simulink library "FuelSystemLibrary"  (R2014b)
settings: Solver=ode45  SolverMode=SingleTasking  StartTime=0.0  StopTime=10.0  RelTol=1e-3
undefined symbols (not defined in the file): BooleanOff, BooleanOn, BoolThreshold, BowserOnPressure, CouplingOffPressure, CouplingOnPressure, DefaultTemp, DiffuserResistance, DiscreteSwitchOff, DiscreteSwitchOn, DiscreteSwitchThreshold, FloatingPressure, FlowNoOverride, FspSamplingPeriod, FuelSpecificHeatCapacity, g, InfiniteFlow, InfiniteMass, InfiniteResistance, InfiniteTime, InfiniteVolume, kpl2kpm3, MaxAValue, MaxBValue, MeterNoReset, MinAValue, MinBValue, NearZeroMass, NearZeroTime, NoError, NominalAValue, NominalBValue, NonRetResistance, NoReset, NullBasePress, PerCycle2PerSec, PerSec2PerCycle, PipeDisconnected, PipeResistance, PumpOnTime, TankFixedMassError, TankInletResistance, TankInstPortStartOffset, TankNoReset, TypicalFuelDensity, ValveClosedPosition, ValveOnResistance, ValveOpenPosition, ValveOpenTime
libraries: FuelSystemLibrary x251, WrightSolverLib x50, simulink x1
(part 2 of 4)

== system FuelSystemLibrary/NRV_V2 ==
  note: No source available downstream,
      | no sink available upstream
  note: NRV: Simulation of Non Return Valve, using WrightSolver diode
      |
      | Revision History -
      | Issue 1.0 - 5th April 2011 - SW - Initial Issue
  BBBrk : FuelSystemLibrary/BBBrk
  BBBrk1 : FuelSystemLibrary/BBBrk1
  BBSrcBrk : FuelSystemLibrary/BBSrcBrk
  Constant2 : Constant  Value=0
  Diode_V2 : WrightSolverLib/Diode_V2
  SinkBrk : FuelSystemLibrary/BBSinkBrk
  Terminator3 : Terminator
  1P : PMIOPort  Tag=PMCPort  Port=1  Side=Left
  2P : PMIOPort  Tag=PMCPort  Port=2  Side=Right
  1BB : PMIOPort  Tag=PMCPort  Port=3  Side=Left
  2BB : PMIOPort  Tag=PMCPort  Port=4  Side=Right
  wires:
  Diode_V2/1 -> Terminator3/1
  Constant2/1 -> Diode_V2/1
  BBBrk1/1 -> SinkBrk/1
  SinkBrk/1 -> BBBrk/1
  BBBrk/1 -> BBSrcBrk/1
  BBSrcBrk/1 -> BBBrk1/1
  connections:
  1P/RConn1 -- Diode_V2/LConn1
  Diode_V2/RConn1 -- 2P/RConn1
  1BB/RConn1 -- BBBrk1/RConn1
  BBBrk/LConn1 -- 2BB/RConn1

== system FuelSystemLibrary/NumInPlug ==
  note: NumInPlug - Plug for numerical interface to tank
      |
      | Revision History -
      | Issue 1.0 - ?? - SW - Initial Issue
      | Issue 1.1 - 28th October 2005 - DR - Added to FSP Generic Library
  BBTerm : FuelSystemLibrary/BBTerm
  Constant : Constant  Value=0
  Terminator8 : Terminator
  Two-Way Connection1 : TwoWayConnection
  1P : PMIOPort  Tag=PMCPort  Port=1  Side=Right
  1BB : PMIOPort  Tag=PMCPort  Port=2  Side=Right
  wires:
  Two-Way Connection1/1 -> Terminator8/1
  Constant/1 -> Two-Way Connection1/1
  connections:
  Two-Way Connection1/RConn1 -- 1P/RConn1
  BBTerm/LConn1 -- 1BB/RConn1

== system FuelSystemLibrary/OFlowIface ==
  note: Translate crude Oflow interface into
      | numerical interface
  Oflow : Inport
  BBBrk : FuelSystemLibrary/BBBrk
  BBStub : FuelSystemLibrary/BBStub
  Demux6 : Demux  Outputs=2
  Terminator8 : Terminator
  Two-Way Connection1 : TwoWayConnection
  P : PMIOPort  Tag=PMCPort  Port=1  Side=Right
  BB : PMIOPort  Tag=PMCPort  Port=2  Side=Right
  wires:
  Demux6/2 -> BBBrk/1  "Info"
  Demux6/1 -> Two-Way Connection1/1  "Mass"
  Oflow/1 -> Demux6/1
  Two-Way Connection1/1 -> Terminator8/1
  BBBrk/1 -> BBStub/1
  connections:
  Two-Way Connection1/RConn1 -- P/RConn1
  BB/RConn1 -- BBBrk/LConn1

== system FuelSystemLibrary/OflowPlug ==
  BBNull : FuelSystemLibrary/BBNull
  Constant2 : Constant  Value=0
  P : Outport
  BB : Outport  Port=2
  wires:
  BBNull/1 -> BB/1
  Constant2/1 -> P/1

== system FuelSystemLibrary/Oriface ==
  C : Inport
  Delay : UnitDelay  InitialCondition=0.0  SampleTime=FspSamplingPeriod
  Delay1 : UnitDelay  InitialCondition=1000000.0  SampleTime=FspSamplingPeriod
  Res : WrightSolverLib/Res
  S-Function : S-Function  FunctionName=OrifaceControlBlockWrapper  EnableBusSupport=off
  2P : PMIOPort  Tag=PMCPort  Port=1  Side=Right
  1P : PMIOPort  Tag=PMCPort  Port=2  Side=Left
  1BB : PMIOPort  Tag=PMCPort  Port=3  Side=Left
  2BB : PMIOPort  Tag=PMCPort  Port=4  Side=Right
  wires:
  Res/1 -> Delay/1
  C/1 -> S-Function/2
  S-Function/1 -> Res/1, Delay1/1
  Delay/1 -> S-Function/1
  Delay1/1 -> S-Function/3
  connections:
  1P/RConn1 -- Res/LConn1
  Res/RConn1 -- 2P/RConn1
  1BB/RConn1 -- 2BB/RConn1

== system FuelSystemLibrary/Outlet ==
  note: outlet
      |
      | Revision History -
      | Issue 1.0 - ?? - SW - Initial Issue
      | Issue 1.1 - 28th October 2005 - DR - Added to FSP Generic Library
  note: Elevate the IO pressures
      | due to head pressures.
  note: We can assume that all tank outlets are connected to
      | pumps, thus ensuring that there can be no backflow
      | into the tank, or outflow if the outlet is not covered.
      |
      | Therefore no diode or cutoff switch, for maximum modelling efficiency.
  HeadPress : Inport
  PipeCovered : Inport  Port=2
  Constant12 : Constant  Value=FlowNoOverride
  I Tap : WrightSolverLib/I Tap
  Term : WrightSolverLib/Term
  Terminator : Terminator
  V : WrightSolverLib/V
  O1P : PMIOPort  Tag=PMCPort  Port=1  Side=Right
  Outflow : Outport
  wires:
  PipeCovered/1 -> Terminator/1
  [OutFlow] -> Outflow/1
  I Tap/1 -> [OutFlow]
  HeadPress/1 -> V/1
  Constant12/1 -> V/2, V/3
  connections:
  Term/RConn1 -- V/LConn1
  I Tap/RConn1 -- O1P/RConn1
  V/RConn1 -- I Tap/LConn1

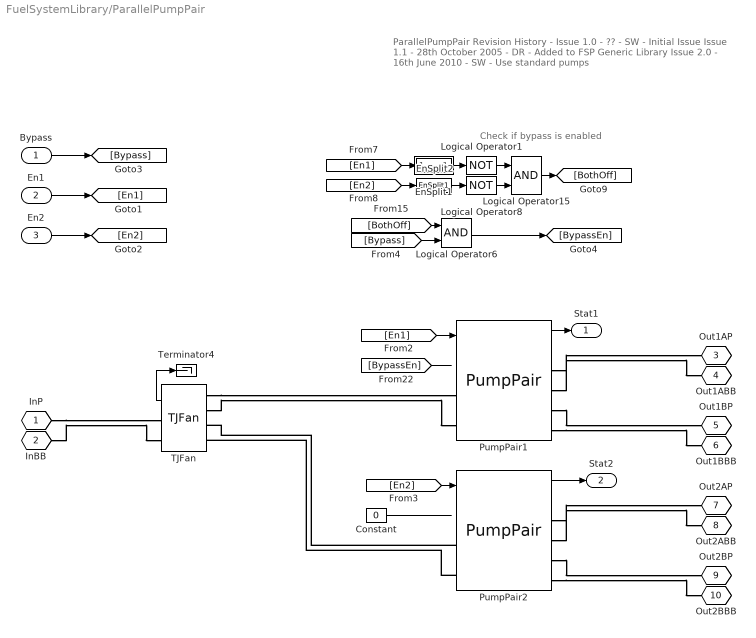
== system FuelSystemLibrary/ParallelPumpPair ==
  note: ParallelPumpPair
      |
      | Revision History -
      | Issue 1.0 - ?? - SW - Initial Issue
      | Issue 1.1 - 28th October 2005 - DR - Added to FSP Generic Library
      | Issue 2.0 - 16th June 2010 - SW - Use standard pumps
  note: Check if bypass is enabled
  Bypass : Inport
  En1 : Inport  Port=2
  En2 : Inport  Port=3
  Constant : Constant  Value=0
  EnSplit1 : Subsystem
  EnSplit2 : FuelSystemLibrary/ParallelPumpPair/EnSplit1
  Logical Operator1 : Logic  Operator=NOT  Inputs=3  AllPortsSameDT=off
  Logical Operator15 : Logic  AllPortsSameDT=off
  Logical Operator6 : Logic  AllPortsSameDT=off
  Logical Operator8 : Logic  Operator=NOT  Inputs=3  AllPortsSameDT=off
  PumpPair1 : FuelSystemLibrary/PumpPair
  PumpPair2 : FuelSystemLibrary/PumpPair
  TJFan : FuelSystemLibrary/TJFan
  Terminator4 : Terminator
  InP : PMIOPort  Tag=PMCPort  Port=1  Side=Left
  InBB : PMIOPort  Tag=PMCPort  Port=2  Side=Left
  Out1AP : PMIOPort  Tag=PMCPort  Port=3  Side=Right
  Out1ABB : PMIOPort  Tag=PMCPort  Port=4  Side=Right
  Out1BP : PMIOPort  Tag=PMCPort  Port=5  Side=Right
  Out1BBB : PMIOPort  Tag=PMCPort  Port=6  Side=Right
  Out2AP : PMIOPort  Tag=PMCPort  Port=7  Side=Right
  Out2ABB : PMIOPort  Tag=PMCPort  Port=8  Side=Right
  Out2BP : PMIOPort  Tag=PMCPort  Port=9  Side=Right
  Out2BBB : PMIOPort  Tag=PMCPort  Port=10  Side=Right
  Stat1 : Outport
  Stat2 : Outport  Port=2
  wires:
  TJFan/1 -> Terminator4/1
  Constant/1 -> ?
  [En1] -> PumpPair1/1
  PumpPair1/1 -> Stat1/1
  PumpPair2/1 -> Stat2/1
  [BypassEn] -> ?
  Bypass/1 -> [Bypass]
  [Bypass] -> Logical Operator6/2
  [BothOff] -> Logical Operator6/1
  Logical Operator15/1 -> [BothOff]
  Logical Operator8/1 -> Logical Operator15/2
  Logical Operator1/1 -> Logical Operator15/1
  EnSplit2/1 -> Logical Operator8/1
  Logical Operator6/1 -> [BypassEn]
  EnSplit1/1(On) -> Logical Operator1/1
  [En1] -> EnSplit1/1(En)
  [En2] -> EnSplit2/1
  En1/1 -> [En1]
  En2/1 -> [En2]
  [En2] -> PumpPair2/1
  connections:
  PumpPair2/LConn2 -- TJFan/LConn4
  PumpPair2/LConn1 -- TJFan/LConn3
  TJFan/LConn2 -- PumpPair1/LConn2
  TJFan/LConn1 -- PumpPair1/LConn1
  InBB/RConn1 -- TJFan/RConn2
  InP/RConn1 -- TJFan/RConn1
  PumpPair2/RConn2 -- Out2ABB/RConn1
  PumpPair2/RConn1 -- Out2AP/RConn1
  PumpPair2/RConn3 -- Out2BP/RConn1
  PumpPair2/RConn4 -- Out2BBB/RConn1
  PumpPair1/RConn1 -- Out1AP/RConn1
  PumpPair1/RConn2 -- Out1ABB/RConn1
  PumpPair1/RConn3 -- Out1BP/RConn1
  PumpPair1/RConn4 -- Out1BBB/RConn1

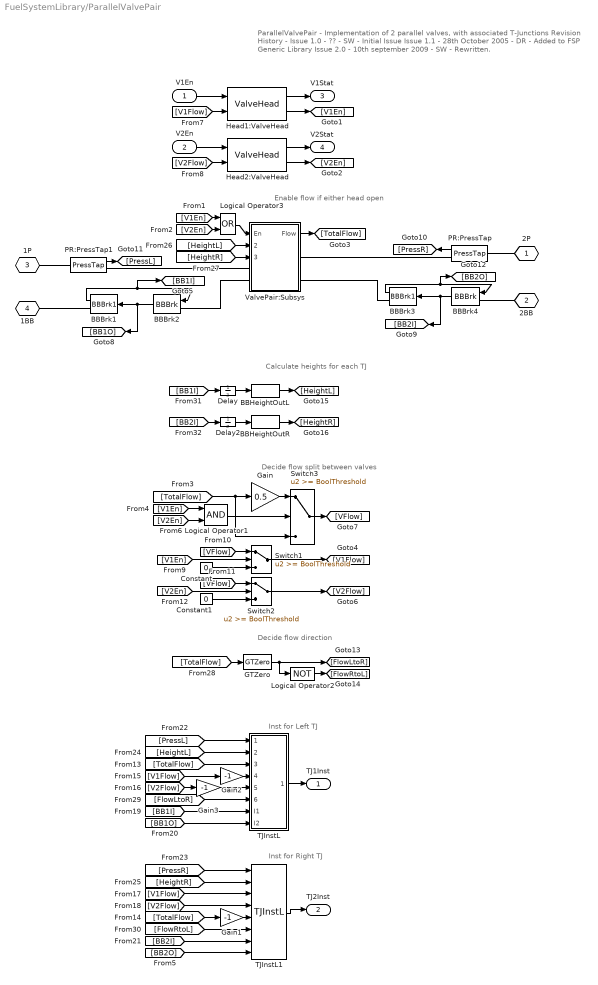
== system FuelSystemLibrary/ParallelValvePair ==
  note: ParallelValvePair - Implementation of 2 parallel valves, with associated T-Junctions
      | Revision History -
      | Issue 1.0 - ?? - SW - Initial Issue
      | Issue 1.1 - 28th October 2005 - DR - Added to FSP Generic Library
      | Issue 2.0 - 10th september 2009 - SW - Rewritten.
  note: Enable flow if either head open
  note: Decide flow split between valves
  note: Inst for Left TJ
  note: Inst for Right TJ
  note: Decide flow direction
  note: Calculate heights for each TJ
  V1En : Inport
  V2En : Inport  Port=2
  BBBrk1 : FuelSystemLibrary/BBBrk1
  BBBrk2 : FuelSystemLibrary/BBBrk
  BBBrk3 : FuelSystemLibrary/BBBrk1
  BBBrk4 : FuelSystemLibrary/BBBrk
  BBHeightOutL : FuelSystemLibrary/BBHeightOut
  BBHeightOutR : FuelSystemLibrary/BBHeightOut
  Constant : Constant  Value=0
  Constant1 : Constant  Value=0
  Delay : UnitDelay  SampleTime=FspSamplingPeriod
  Delay2 : UnitDelay  SampleTime=FspSamplingPeriod
  GTZero : FuelSystemLibrary/GTZero
  Gain : Gain  Gain=0.5  SaturateOnIntegerOverflow=on  OutDataTypeStr=Inherit: Same as input  ParamDataTypeStr=Inherit: Same as input
  Gain1 : Gain  Gain=-1  SaturateOnIntegerOverflow=on  OutDataTypeStr=Inherit: Same as input  ParamDataTypeStr=Inherit: Same as input
  Gain2 : Gain  Gain=-1  SaturateOnIntegerOverflow=on  OutDataTypeStr=Inherit: Same as input  ParamDataTypeStr=Inherit: Same as input
  Gain3 : Gain  Gain=-1  SaturateOnIntegerOverflow=on  OutDataTypeStr=Inherit: Same as input  ParamDataTypeStr=Inherit: Same as input
  Head1:ValveHead : FuelSystemLibrary/ValveHead
  Head2:ValveHead : FuelSystemLibrary/ValveHead
  Logical Operator1 : Logic  AllPortsSameDT=off
  Logical Operator2 : Logic  Operator=NOT  AllPortsSameDT=off
  Logical Operator3 : Logic  Operator=OR  AllPortsSameDT=off
  PR:PressTap : FuelSystemLibrary/PressTap
  PR:PressTap1 : FuelSystemLibrary/PressTap
  Switch1 : Switch  Threshold=BoolThreshold  SaturateOnIntegerOverflow=on  InputSameDT=on
  Switch2 : Switch  Threshold=BoolThreshold  SaturateOnIntegerOverflow=on  InputSameDT=on
  Switch3 : Switch  Threshold=BoolThreshold  SaturateOnIntegerOverflow=on  InputSameDT=on
  TJInstL : Subsystem
  TJInstL1 : FuelSystemLibrary/ParallelValvePair/TJInstL
  ValvePair:Subsys : Subsystem
  2P : PMIOPort  Tag=PMCPort  Port=1  Side=Right
  2BB : PMIOPort  Tag=PMCPort  Port=2  Side=Right
  1P : PMIOPort  Tag=PMCPort  Port=3  Side=Left
  1BB : PMIOPort  Tag=PMCPort  Port=4  Side=Left
  TJ1Inst : Outport
  TJ2Inst : Outport  Port=2
  V1Stat : Outport  Port=3
  V2Stat : Outport  Port=4
  wires:
  [HeightL] -> TJInstL/2(Height)
  BBBrk3/1 -> [BB2O], BBBrk4/1
  BBBrk4/1 -> [BB2I], BBBrk3/1
  BBBrk1/1 -> [BB1I], BBBrk2/1
  BBBrk2/1 -> [BB1O], BBBrk1/1
  V1En/1 -> Head1:ValveHead/1
  V2En/1 -> Head2:ValveHead/1
  Head1:ValveHead/1 -> V1Stat/1
  Head2:ValveHead/1 -> V2Stat/1
  Head1:ValveHead/2 -> [V1En]
  Head2:ValveHead/2 -> [V2En]
  Logical Operator3/1 -> ValvePair:Subsys/1(En)
  [V1En] -> Logical Operator3/1
  [V2En] -> Logical Operator3/2
  ValvePair:Subsys/1(Flow) -> [TotalFlow]
  [TotalFlow] -> Switch3/3, Gain/1
  [V1Flow] -> Head1:ValveHead/2
  [V2Flow] -> Head2:ValveHead/2
  [V1En] -> Logical Operator1/1
  [V2En] -> Logical Operator1/2
  Logical Operator1/1 -> Switch3/2
  Gain/1 -> Switch3/1
  Switch3/1 -> [VFlow]
  [V1En] -> Switch1/2
  Constant/1 -> Switch1/3
  [VFlow] -> Switch1/1
  Switch1/1 -> [V1Flow]
  [V2En] -> Switch2/2
  Constant1/1 -> Switch2/3
  [VFlow] -> Switch2/1
  Switch2/1 -> [V2Flow]
  TJInstL/1(Inst) -> TJ1Inst/1
  [TotalFlow] -> TJInstL/3(Flow1)
  [TotalFlow] -> Gain1/1
  [V1Flow] -> Gain2/1
  [V2Flow] -> Gain3/1
  Gain2/1 -> TJInstL/4(Flow2)
  Gain3/1 -> TJInstL/5(Flow3)
  [BB2I] -> TJInstL1/7
  [BB1I] -> TJInstL/7(I1)
  [PressL] -> TJInstL/1(Press)
  TJInstL1/1 -> TJ2Inst/1
  [BB1O] -> TJInstL/8(I2)
  [BB2O] -> TJInstL1/8
  Gain1/1 -> TJInstL1/5
  [V1Flow] -> TJInstL1/3
  [V2Flow] -> TJInstL1/4
  [TotalFlow] -> GTZero/1
  GTZero/1 -> [FlowLtoR], Logical Operator2/1
  Logical Operator2/1 -> [FlowRtoL]
  [FlowLtoR] -> TJInstL/6(I1nI2)
  [FlowRtoL] -> TJInstL1/6
  [PressR] -> TJInstL1/1
  [HeightR] -> TJInstL1/2
  [HeightL] -> ValvePair:Subsys/2(HeightL)
  [HeightR] -> ValvePair:Subsys/3(HeightR)
  [BB1I] -> Delay/1
  [BB2I] -> Delay2/1
  Delay/1 -> BBHeightOutL/1
  Delay2/1 -> BBHeightOutR/1
  BBHeightOutR/1 -> [HeightR]
  BBHeightOutL/1 -> [HeightL]
  PR:PressTap1/1 -> [PressL]
  PR:PressTap/1 -> [PressR]
  connections:
  ValvePair:Subsys/RConn2 -- BBBrk3/RConn1
  BBBrk4/LConn1 -- 2BB/RConn1
  BBBrk2/LConn1 -- ValvePair:Subsys/LConn2
  1BB/RConn1 -- BBBrk1/RConn1
  PR:PressTap1/RConn1 -- ValvePair:Subsys/LConn1
  1P/RConn1 -- PR:PressTap1/LConn1
  2P/RConn1 -- PR:PressTap/LConn1
  ValvePair:Subsys/RConn1 -- PR:PressTap/RConn1

== system FuelSystemLibrary/Pipe ==
  Constant1 : Constant  Value=PipeResistance
  Res : WrightSolverLib/Res
  Terminator8 : Terminator
  1P : PMIOPort  Tag=PMCPort  Port=1  Side=Left
  1BB : PMIOPort  Tag=PMCPort  Port=2  Side=Left
  2P : PMIOPort  Tag=PMCPort  Port=3  Side=Right
  2BB : PMIOPort  Tag=PMCPort  Port=4  Side=Right
  wires:
  Constant1/1 -> Res/1
  Res/1 -> Terminator8/1
  connections:
  1BB/RConn1 -- 2BB/RConn1
  1P/RConn1 -- Res/LConn1
  Res/RConn1 -- 2P/RConn1

== system FuelSystemLibrary/PipeMass ==
  Inst : Inport
  Demux4 : Demux  Outputs=9
  Terminator{1..2,4,7,16..19} (8 alike) : Terminator
  Mass : Outport
  wires:
  Demux4/1 -> Terminator7/1  "Mass"
  Demux4/9 -> Terminator19/1  "CG_Vert"
  Demux4/8 -> Terminator18/1  "Inflow2"
  Demux4/7 -> Terminator17/1  "Height2"
  Demux4/6 -> Terminator2/1  "Inflow1"
  Demux4/5 -> Terminator1/1  "Height1"
  Demux4/4 -> Terminator16/1  "BVal"
  Demux4/3 -> Terminator4/1  "AVal"
  Demux4/2 -> Mass/1  "Temp"
  Inst/1 -> Demux4/1

== system FuelSystemLibrary/Port Press ==
  note: Revision History -
      | Issue 1.0 - 11th November 2009 - SW - Initial Issue
  note: Calculate head pressure at selected port
  Inst : Inport
  Port : Inport  Port=2
  Constant1 : Constant  Value=TankInstPortStartOffset
  Constant2 : Constant  Value=g
  Demux4 : Demux  Outputs=20
  Multiport Switch : MultiPortSwitch  DataPortOrder=Zero-based contiguous  Inputs=5  zeroidx=on  SaturateOnIntegerOverflow=on
  Product : Product  Inputs=3  SaturateOnIntegerOverflow=on  OutDataTypeStr=Inherit: Same as first input
  Sum1 : Sum  Inputs=|+-  SaturateOnIntegerOverflow=on
  Sum2 : Sum  Inputs=|+-  SaturateOnIntegerOverflow=on
  Temp2Density : FuelSystemLibrary/Temp2Density
  Terminator{2..10,16..17} (11 alike) : Terminator
  Press : Outport
  wires:
  Demux4/13 -> Terminator6/1
  Demux4/14 -> Terminator10/1
  Demux4/15 -> Terminator5/1
  Inst/1 -> Demux4/1
  Demux4/1 -> Terminator16/1  "MaxVolume"
  Demux4/2 -> Terminator4/1  "Mass"
  Demux4/3 -> Terminator17/1  "Volume"
  Demux4/4 -> [SurfaceHeight]  "SurfaceHeight"
  Demux4/5 -> Terminator2/1  "InFlow"
  Demux4/6 -> Temp2Density/1  "Temp"
  Demux4/7 -> Temp2Density/2  "AValue"
  Demux4/8 -> Temp2Density/3  "BValue"
  Demux4/9 -> Terminator7/1
  Demux4/10 -> Terminator8/1
  Demux4/11 -> Terminator9/1
  Temp2Density/1 -> Product/1
  Demux4/12 -> Terminator3/1
  Constant2/1 -> Product/2
  Product/1 -> Press/1
  Demux4/16 -> Multiport Switch/2  "Inlet1Height"
  Demux4/17 -> Multiport Switch/3  "Inlet2Height"
  Demux4/18 -> Multiport Switch/4  "Inlet3Height"
  Demux4/19 -> Multiport Switch/5  "Outlet1Height"
  Demux4/20 -> Multiport Switch/6  "Outlet2Height"
  Port/1 -> Sum2/1
  Constant1/1 -> Sum2/2
  Sum2/1 -> [PortIndex]
  [PortIndex] -> Multiport Switch/1
  Multiport Switch/1 -> Sum1/2
  Sum1/1 -> Product/3
  [SurfaceHeight] -> Sum1/1

== system FuelSystemLibrary/PressSwitch ==
  note: Pressure Switch
      |
      | Revision History -
      | Issue 1.0 - ?? - SW - Initial Issue
      | Issue 1.1 - 28th October 2005 - DR - Added to FSP Generic Library
  En : Inport
  OnP : Inport  Port=2
  OffP : Inport  Port=3
  BBI1 : FuelSystemLibrary/BBI1
  BBI2 : FuelSystemLibrary/BBI1
  PressSwitchCore : FuelSystemLibrary/PressSwitchCore
  PressTap : FuelSystemLibrary/PressTap
  1P : PMIOPort  Tag=PMCPort  Port=1  Side=Left
  1BB : PMIOPort  Tag=PMCPort  Port=2  Side=Left
  2P : PMIOPort  Tag=PMCPort  Port=3  Side=Right
  2BB : PMIOPort  Tag=PMCPort  Port=4  Side=Right
  Stat : Outport
  wires:
  BBI2/1 -> PressSwitchCore/6
  BBI1/1 -> PressSwitchCore/5
  OnP/1 -> PressSwitchCore/2
  PressTap/1 -> PressSwitchCore/4
  OffP/1 -> PressSwitchCore/3
  PressSwitchCore/1 -> Stat/1
  En/1 -> PressSwitchCore/1
  connections:
  BBI2/LConn1 -- 2BB/RConn1
  1BB/RConn1 -- BBI1/LConn1
  BBI1/RConn1 -- BBI2/RConn1
  PressTap/LConn1 -- 1P/RConn1
  PressTap/RConn1 -- 2P/RConn1

== system FuelSystemLibrary/PressSwitchCore ==
  note: Assume that the inlet base
      | pressure is right base pressure
      | for this component
  note: Read zero pressure
      | if switch is isolated
      | or pump is off
  note: Output Hi for
      | low pressure
  note: Generate -1/0/1, depending on
      | whether below, betweenor above
      | thresholds
  note: Pressure Switch Core
      |
      | Revision History -
      | Issue 1.0 - ?? - SW - Initial Issue
      | Issue 1.1 - 28th October 2005 - DR - Added to FSP Generic Library
  note: This logic could be removed,
      | as replaced by
      | FloatingPressure detection
  En : Inport
  OnP : Inport  Port=2
  OffP : Inport  Port=3
  1P : Inport  Port=4
  1I : Inport  Port=5
  1O : Inport  Port=6
  BBBasePOut : FuelSystemLibrary/BBBasePOut
  BBSrcAvailOut1 : FuelSystemLibrary/BBSrcAvailOut
  BBSrcAvailOut2 : FuelSystemLibrary/BBSrcAvailOut
  Compare To Constant : simulink/Logic and Bit Operations/Compare To Constant  relop=~=  const=FloatingPressure  OutDataTypeStr=uint8  ZeroCross=off
  Data Type Conversion : DataTypeConversion  OutDataTypeStr=double
  Logical Operator : Logic  Operator=NOT  AllPortsSameDT=off
  Logical Operator1 : Logic  Operator=OR  AllPortsSameDT=off
  Logical Operator2 : Logic  Inputs=4  AllPortsSameDT=off
  Relational Operator : RelationalOperator  Operator=>
  Relational Operator1 : RelationalOperator  Operator=<
  Sum : Sum  Inputs=|+-  SaturateOnIntegerOverflow=on
  Sum1 : Sum  Inputs=|+-  SaturateOnIntegerOverflow=on
  Stat : Outport
  wires:
  1P/1 -> Sum1/1, Compare To Constant/1
  BBBasePOut/1 -> Sum1/2
  [En] -> Logical Operator2/4
  En/1 -> [En]
  Logical Operator1/1 -> Logical Operator2/3
  Logical Operator2/1 -> Logical Operator/1
  Sum/1 -> Logical Operator2/2
  BBSrcAvailOut2/1 -> Logical Operator1/2
  BBSrcAvailOut1/1 -> Logical Operator1/1
  Logical Operator/1 -> Data Type Conversion/1
  OffP/1 -> [OffPress]
  Relational Operator1/1 -> Sum/2
  Relational Operator/1 -> Sum/1
  [OffPress] -> Relational Operator1/2
  [OnPress] -> Relational Operator/2
  OnP/1 -> [OnPress]
  Sum1/1 -> Relational Operator1/1, Relational Operator/1
  1O/1 -> BBSrcAvailOut2/1
  1I/1 -> BBSrcAvailOut1/1, BBBasePOut/1
  Compare To Constant/1 -> Logical Operator2/1
  Data Type Conversion/1 -> Stat/1

== system FuelSystemLibrary/PressTap ==
  V Tap : WrightSolverLib/V Tap
  1 : PMIOPort  Tag=PMCPort  Port=1  Side=Left
  2 : PMIOPort  Tag=PMCPort  Port=2  Side=Right
  Press : Outport
  wires:
  V Tap/1 -> Press/1
  connections:
  1/RConn1 -- V Tap/LConn1
  V Tap/RConn1 -- 2/RConn1

== system FuelSystemLibrary/PressureValve ==
  note: Pressure Valve - requires Control Enable signal and
      | active forward pressure to open
  En : Inport
  1SinkAvail : FuelSystemLibrary/SinkAvail
  1SrcAvail : FuelSystemLibrary/SrcAvail
  2SinkAvail : FuelSystemLibrary/SinkAvail
  2SrcAvail : FuelSystemLibrary/SrcAvail
  Constant6 : Constant  Value=0
  Delay : UnitDelay  InitialCondition=InfiniteResistance  SampleTime=-1
  Demux : Demux  Outputs=3
  Logical Operator : Logic  AllPortsSameDT=off
  Logical Operator1 : Logic  AllPortsSameDT=off
  Logical Operator2 : Logic  Operator=OR  AllPortsSameDT=off
  Mux : Mux  Inputs=3
  RS: Valve1Ip : FuelSystemLibrary/Valve1Ip
  Switch : Switch  Criteria=u2 ~= 0  SaturateOnIntegerOverflow=on
  1P : PMIOPort  Tag=PMCPort  Port=1  Side=Left
  1BB : PMIOPort  Tag=PMCPort  Port=2  Side=Left
  2P : PMIOPort  Tag=PMCPort  Port=3  Side=Right
  2BB : PMIOPort  Tag=PMCPort  Port=4  Side=Right
  Stat : Outport
  wires:
  [PathEn] -> Switch/2
  Constant6/1 -> Switch/3
  Logical Operator2/1 -> Delay/1
  Logical Operator1/1 -> Logical Operator2/2
  Logical Operator/1 -> Logical Operator2/1
  [SnkA1] -> Logical Operator1/2
  [SrcA2] -> Logical Operator1/1
  [SnkA2] -> Logical Operator/2
  [SrcA1] -> Logical Operator/1
  Switch/1 -> Mux/1
  Mux/1 -> [En]
  Demux/2 -> Mux/2  "SwitchTime"
  Demux/1 -> Switch/1  "OnEn"
  En/1 -> Demux/1
  Demux/3 -> Mux/3  "ErrorCode"
  [En] -> RS: Valve1Ip/1
  RS: Valve1Ip/1 -> Stat/1
  1SrcAvail/1 -> [SrcA1]
  1SinkAvail/1 -> [SnkA1]
  2SinkAvail/1 -> [SnkA2]
  2SrcAvail/1 -> [SrcA2]
  Delay/1 -> [PathEn]
  connections:
  1P/RConn1 -- RS: Valve1Ip/LConn1
  1SrcAvail/RConn1 -- 1SinkAvail/LConn1
  2SrcAvail/RConn1 -- 2SinkAvail/LConn1
  2SrcAvail/LConn1 -- 2BB/RConn1
  RS: Valve1Ip/RConn2 -- 2SinkAvail/RConn1
  2P/RConn1 -- RS: Valve1Ip/RConn1
  1BB/RConn1 -- 1SrcAvail/LConn1
  1SinkAvail/RConn1 -- RS: Valve1Ip/LConn2

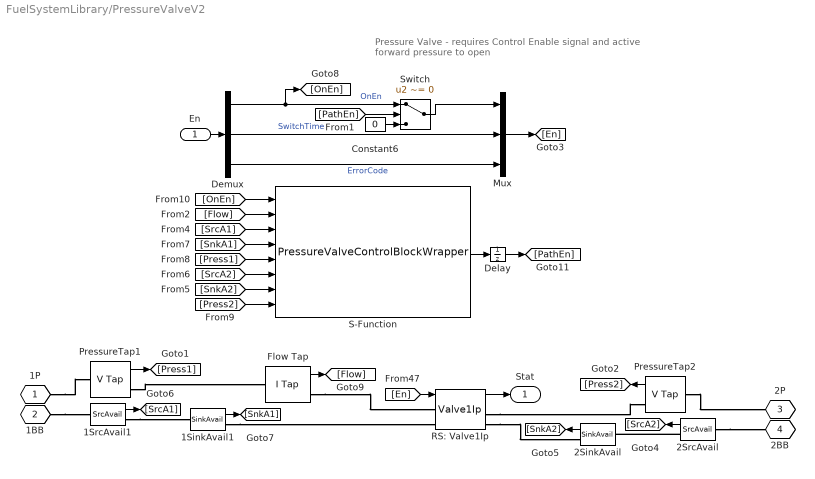
== system FuelSystemLibrary/PressureValveV2 ==
  note: Pressure Valve - requires Control Enable signal and
      | active forward pressure to open
  En : Inport
  1SinkAvail1 : FuelSystemLibrary/SinkAvail
  1SrcAvail1 : FuelSystemLibrary/SrcAvail
  2SinkAvail : FuelSystemLibrary/SinkAvail
  2SrcAvail : FuelSystemLibrary/SrcAvail
  Constant6 : Constant  Value=0
  Delay : UnitDelay  InitialCondition=InfiniteResistance  SampleTime=-1
  Demux : Demux  Outputs=3
  Flow Tap : WrightSolverLib/I Tap
  Mux : Mux  Inputs=3
  PressureTap1 : WrightSolverLib/V Tap
  PressureTap2 : WrightSolverLib/V Tap
  RS: Valve1Ip : FuelSystemLibrary/Valve1Ip
  S-Function : S-Function  FunctionName=PressureValveControlBlockWrapper  EnableBusSupport=off
  Switch : Switch  Criteria=u2 ~= 0  SaturateOnIntegerOverflow=on
  1P : PMIOPort  Tag=PMCPort  Port=1  Side=Left
  1BB : PMIOPort  Tag=PMCPort  Port=2  Side=Left
  2P : PMIOPort  Tag=PMCPort  Port=3  Side=Right
  2BB : PMIOPort  Tag=PMCPort  Port=4  Side=Right
  Stat : Outport
  wires:
  RS: Valve1Ip/1 -> Stat/1
  [En] -> RS: Valve1Ip/1
  Demux/3 -> Mux/3  "ErrorCode"
  En/1 -> Demux/1
  Demux/1 -> Switch/1, [OnEn]  "OnEn"
  Demux/2 -> Mux/2  "SwitchTime"
  Mux/1 -> [En]
  Switch/1 -> Mux/1
  Constant6/1 -> Switch/3
  [PathEn] -> Switch/2
  PressureTap1/1 -> [Press1]
  PressureTap2/1 -> [Press2]
  2SinkAvail/1 -> [SnkA2]
  2SrcAvail/1 -> [SrcA2]
  S-Function/1 -> Delay/1
  1SrcAvail1/1 -> [SrcA1]
  1SinkAvail1/1 -> [SnkA1]
  Delay/1 -> [PathEn]
  [OnEn] -> S-Function/1
  [Flow] -> S-Function/2
  [SrcA1] -> S-Function/3
  [SnkA1] -> S-Function/4
  [Press1] -> S-Function/5
  [SrcA2] -> S-Function/6
  [SnkA2] -> S-Function/7
  [Press2] -> S-Function/8
  Flow Tap/1 -> [Flow]
  connections:
  1P/RConn1 -- PressureTap1/LConn1
  PressureTap2/LConn1 -- 2P/RConn1
  RS: Valve1Ip/RConn1 -- PressureTap2/RConn1
  RS: Valve1Ip/RConn2 -- 2SinkAvail/RConn1
  2SrcAvail/RConn1 -- 2SinkAvail/LConn1
  1SrcAvail1/RConn1 -- 1SinkAvail1/LConn1
  1SinkAvail1/RConn1 -- RS: Valve1Ip/LConn2
  1BB/RConn1 -- 1SrcAvail1/LConn1
  2SrcAvail/LConn1 -- 2BB/RConn1
  PressureTap1/RConn1 -- Flow Tap/LConn1
  Flow Tap/RConn1 -- RS: Valve1Ip/LConn1

== system FuelSystemLibrary/Proportional2Mix ==
  note: Mix 2 incoming signals in proportion to their masses
      |
      | Revision History -
      | Issue 1.0 - ?? - SW - Initial Issue
      | Issue 1.1 - 28th October 2005 - DR - Added to FSP Generic Library and Includes fix for Temperature Calculation for Near-Zero flow
      | Issue 2.0 - 15th June 2010 - Wrapper for valid-flag version
      | Issue 2.1 - 23rd June 2010 - SW - Functionality moved to S-function
  Sig1 : Inport
  Mass1 : Inport  Port=2
  Sig2 : Inport  Port=3
  Mass2 : Inport  Port=4
  S-Function : S-Function  FunctionName=ProportionalMixBlockWrapper  EnableBusSupport=off
  Terminator : Terminator
  Sig : Outport
  wires:
  Sig1/1 -> S-Function/1
  Mass1/1 -> S-Function/2
  Sig2/1 -> S-Function/3
  Mass2/1 -> S-Function/4
  S-Function/1 -> Sig/1
  S-Function/2 -> Terminator/1

== system FuelSystemLibrary/Proportional2MixValid ==
  note: Mix 2 incoming signals in proportion to their masses, with validity signal
      |
      | Revision History -
      | Issue 1.0 - 11th November 2009 - SW - Initial Issue
      | Issue 2.0 - 16th June 2010 - SW - Functionality moved to S-function
  Sig1 : Inport
  Mass1 : Inport  Port=2
  Sig2 : Inport  Port=3
  Mass2 : Inport  Port=4
  S-Function : S-Function  FunctionName=ProportionalMixBlockWrapper  EnableBusSupport=off
  Sig : Outport
  Valid : Outport  Port=2
  wires:
  Sig1/1 -> S-Function/1
  Mass1/1 -> S-Function/2
  Sig2/1 -> S-Function/3
  Mass2/1 -> S-Function/4
  S-Function/1 -> Sig/1
  S-Function/2 -> Valid/1

== system FuelSystemLibrary/Proportional3Mix ==
  note: Mix 3 incoming signals in proportion to their masses
      |
      | Revision History -
      | Issue 1.0 - ?? - SW - Initial Issue
      | Issue 1.1 - 28th October 2005 - DR - Added to FSP Generic Library
      | Issue 2.0 - 16th June 2010 - SW - Functionality moved to S-function
  Sig1 : Inport
  Mass1 : Inport  Port=2
  Sig2 : Inport  Port=3
  Mass2 : Inport  Port=4
  Sig3 : Inport  Port=5
  Mass3 : Inport  Port=6
  Mux : Mux  Inputs=2
  S-Function1 : S-Function  FunctionName=ProportionalMixBlockWrapper  EnableBusSupport=off
  S-Function2 : S-Function  FunctionName=ProportionalMixBlockWrapper  EnableBusSupport=off
  Saturation : Saturate  UpperLimit=InfiniteFlow  LowerLimit=0
  Saturation1 : Saturate  UpperLimit=InfiniteFlow  LowerLimit=0
  Scope : Scope
  Sum : Sum  Inputs=|++  SaturateOnIntegerOverflow=on  InputSameDT=on  OutDataTypeStr=Inherit: Same as first input
  Terminator : Terminator
  Terminator1 : Terminator
  Sig : Outport
  wires:
  Sig1/1 -> S-Function1/1
  Mass1/1 -> S-Function1/2, Saturation/1, Mux/1
  Sig2/1 -> S-Function1/3
  Mass2/1 -> S-Function1/4, Saturation1/1, Mux/2
  Sum/1 -> S-Function2/2
  Sig3/1 -> S-Function2/3
  Mass3/1 -> S-Function2/4
  Saturation/1 -> Sum/1
  Saturation1/1 -> Sum/2
  S-Function1/1 -> S-Function2/1
  S-Function1/2 -> Terminator/1
  S-Function2/2 -> Terminator1/1
  S-Function2/1 -> Sig/1
  Mux/1 -> Scope/1

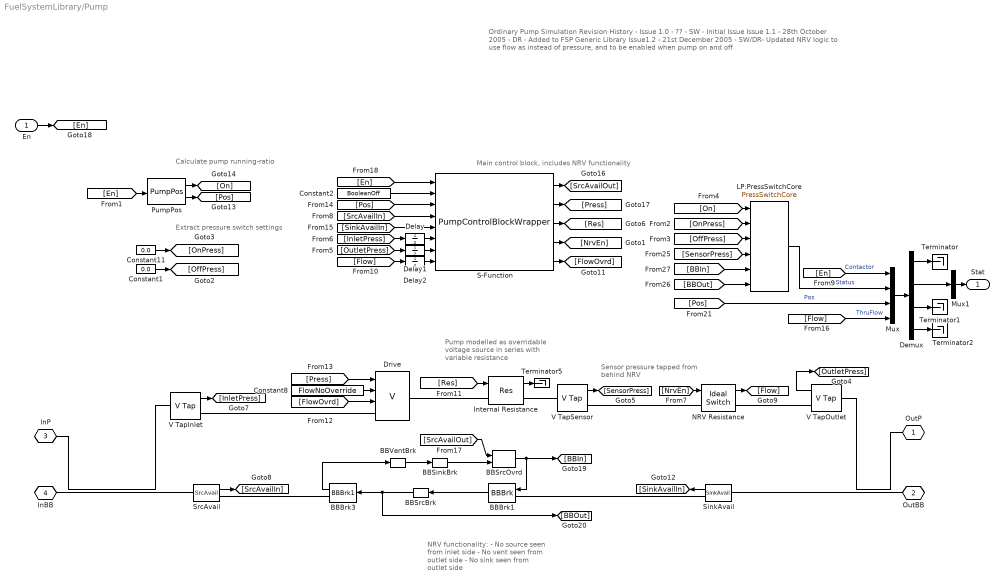
== system FuelSystemLibrary/Pump ==
  note: NRV functionality:
      | - No source seen from inlet side
      | - No vent seen from outlet side
      | - No sink seen from outlet side
  note: Sensor pressure tapped
      | from behind NRV
  note: Main control block, includes NRV functionality
  note: Extract pressure switch settings
  note: Calculate pump running-ratio
  note: Pump modelled as
      | overridable
      | voltage source
      | in series with
      | variable resistance
  note: Ordinary Pump Simulation
      |
      | Revision History -
      | Issue 1.0 - ?? - SW - Initial Issue
      | Issue 1.1 - 28th October 2005 - DR - Added to FSP Generic Library
      | Issue1.2 - 21st December 2005 - SW/DR- Updated NRV logic to use flow as instead of pressure,
      | and to be enabled when pump on and off
  En : Inport
  BBBrk1 : FuelSystemLibrary/BBBrk
  BBBrk3 : FuelSystemLibrary/BBBrk1
  BBSinkBrk : FuelSystemLibrary/BBSinkBrk
  BBSrcBrk : FuelSystemLibrary/BBSrcBrk
  BBSrcOvrd : FuelSystemLibrary/BBSrcOvrd
  BBVentBrk : FuelSystemLibrary/BBVentBrk
  Constant1 : Constant  Value=0.0
  Constant11 : Constant  Value=0.0
  Constant2 : Constant  Value=BooleanOff
  Constant8 : Constant  Value=FlowNoOverride
  Delay : UnitDelay  SampleTime=-1
  Delay1 : UnitDelay  SampleTime=-1
  Delay2 : UnitDelay  SampleTime=-1
  Demux : Demux
  Drive : WrightSolverLib/V
  Internal Resistance : WrightSolverLib/Res
  LP:PressSwitchCore : FuelSystemLibrary/PressSwitchCore
  Mux : Mux
  Mux1 : Mux  Inputs=[1]
  NRV Resistance : WrightSolverLib/Ideal Switch  OnResistance=0
  PumpPos : FuelSystemLibrary/PumpPos
  S-Function : S-Function  FunctionName=PumpControlBlockWrapper  EnableBusSupport=off
  SinkAvail : FuelSystemLibrary/SinkAvail
  SrcAvail : FuelSystemLibrary/SrcAvail
  Terminator{,1..2,5} (4 alike) : Terminator
  V TapInlet : WrightSolverLib/V Tap
  V TapOutlet : WrightSolverLib/V Tap
  V TapSensor : WrightSolverLib/V Tap
  OutP : PMIOPort  Tag=PMCPort  Port=1  Side=Right
  OutBB : PMIOPort  Tag=PMCPort  Port=2  Side=Right
  InP : PMIOPort  Tag=PMCPort  Port=3  Side=Left
  InBB : PMIOPort  Tag=PMCPort  Port=4  Side=Left
  Stat : Outport
  wires:
  S-Function/5 -> [FlowOvrd]
  BBBrk1/1 -> BBSrcBrk/1
  BBSrcBrk/1 -> [BBOut], BBBrk3/1
  [NrvEn] -> NRV Resistance/1
  NRV Resistance/1 -> [Flow]
  En/1 -> [En]
  Constant8/1 -> Drive/2
  [FlowOvrd] -> Drive/3
  Delay2/1 -> S-Function/8
  [SrcAvailIn] -> S-Function/4
  SinkAvail/1 -> [SinkAvailIn]
  [Pos] -> S-Function/3
  [Press] -> Drive/1
  [Res] -> Internal Resistance/1
  S-Function/4 -> [NrvEn]
  S-Function/3 -> [Res]
  S-Function/2 -> [Press]
  S-Function/1 -> [SrcAvailOut]
  Delay1/1 -> S-Function/7
  [Flow] -> Delay2/1
  Delay/1 -> S-Function/6
  [OutletPress] -> Delay1/1
  [SinkAvailIn] -> S-Function/5
  [InletPress] -> Delay/1
  Constant2/1 -> S-Function/2
  [En] -> S-Function/1
  PumpPos/1 -> [On]
  PumpPos/2 -> [Pos]
  [SrcAvailOut] -> BBSrcOvrd/1
  BBSinkBrk/1 -> BBSrcOvrd/2
  BBVentBrk/1 -> BBSinkBrk/1
  SrcAvail/1 -> [SrcAvailIn]
  BBBrk3/1 -> BBVentBrk/1
  BBSrcOvrd/1 -> [BBIn], BBBrk1/1
  V TapInlet/1 -> [InletPress]
  Internal Resistance/1 -> Terminator5/1
  [En] -> PumpPos/1
  Constant1/1 -> [OffPress]
  Constant11/1 -> [OnPress]
  [En] -> Mux/1  "Contactor"
  Mux/1 -> Demux/1
  LP:PressSwitchCore/1 -> Mux/2  "Status"
  [Pos] -> Mux/3  "Pos"
  [SensorPress] -> LP:PressSwitchCore/4
  [On] -> LP:PressSwitchCore/1
  [OnPress] -> LP:PressSwitchCore/2
  [OffPress] -> LP:PressSwitchCore/3
  [BBOut] -> LP:PressSwitchCore/6
  [BBIn] -> LP:PressSwitchCore/5
  [Flow] -> Mux/4  "ThruFlow"
  V TapSensor/1 -> [SensorPress]
  V TapOutlet/1 -> [OutletPress]
  Demux/1 -> Terminator/1
  Demux/4 -> Terminator2/1
  Demux/3 -> Terminator1/1
  Demux/2 -> Mux1/1
  Mux1/1 -> Stat/1
  connections:
  InP/RConn1 -- V TapInlet/LConn1
  SinkAvail/LConn1 -- OutBB/RConn1
  BBBrk1/LConn1 -- SinkAvail/RConn1
  Internal Resistance/RConn1 -- V TapSensor/LConn1
  Drive/RConn1 -- Internal Resistance/LConn1
  InBB/RConn1 -- SrcAvail/LConn1
  V TapInlet/RConn1 -- Drive/LConn1
  SrcAvail/RConn1 -- BBBrk3/RConn1
  V TapSensor/RConn1 -- NRV Resistance/LConn1
  NRV Resistance/RConn1 -- V TapOutlet/RConn1
  V TapOutlet/LConn1 -- OutP/RConn1

== system FuelSystemLibrary/PumpPair ==
  En1 : Inport
  En2 : Inport  Port=2
  "PumpA : Pump" : FuelSystemLibrary/Pump
  "PumpB : Pump" : FuelSystemLibrary/Pump
  TJFan : FuelSystemLibrary/TJFan
  Terminator4 : Terminator
  InP : PMIOPort  Tag=PMCPort  Port=1  Side=Left
  InBB : PMIOPort  Tag=PMCPort  Port=2  Side=Left
  OutAP : PMIOPort  Tag=PMCPort  Port=3  Side=Right
  OutABB : PMIOPort  Tag=PMCPort  Port=4  Side=Right
  OutBP : PMIOPort  Tag=PMCPort  Port=5  Side=Right
  OutBBB : PMIOPort  Tag=PMCPort  Port=6  Side=Right
  Stat1 : Outport
  Stat2 : Outport  Port=2
  wires:
  "PumpB : Pump"/1 -> Stat2/1
  "PumpA : Pump"/1 -> Stat1/1
  En2/1 -> "PumpB : Pump"/1
  En1/1 -> "PumpA : Pump"/1
  TJFan/1 -> Terminator4/1
  connections:
  "PumpA : Pump"/RConn2 -- OutABB/RConn1
  "PumpA : Pump"/RConn1 -- OutAP/RConn1
  InP/RConn1 -- TJFan/RConn1
  InBB/RConn1 -- TJFan/RConn2
  TJFan/LConn3 -- "PumpB : Pump"/LConn1
  TJFan/LConn4 -- "PumpB : Pump"/LConn2
  "PumpB : Pump"/RConn1 -- OutBP/RConn1
  "PumpB : Pump"/RConn2 -- OutBBB/RConn1
  TJFan/LConn1 -- "PumpA : Pump"/LConn1
  TJFan/LConn2 -- "PumpA : Pump"/LConn2

== system FuelSystemLibrary/PumpPos ==
  note: Pump Speed Simulation
  En : Inport
  Constant1 : Constant  Value=PumpOnTime
  Gain : Gain  Gain=-1  SaturateOnIntegerOverflow=on  OutDataTypeStr=Inherit: Same as input  ParamDataTypeStr=Inherit: Same as input
  Math Function : Math  Operator=reciprocal  SaturateOnIntegerOverflow=on
  Prevent div-by-zero : Saturate  UpperLimit=InfiniteTime  LowerLimit=NearZeroTime
  Switch1 : Switch  Threshold=DiscreteSwitchThreshold  SaturateOnIntegerOverflow=on  InputSameDT=on
  ZeroOrder Integrator : FuelSystemLibrary/ZeroOrderIntegrator
  PumpOn : Outport
  Pos : Outport  Port=2
  wires:
  ZeroOrder Integrator/1 -> Pos/1
  Switch1/1 -> ZeroOrder Integrator/1  "UnitSlewRate"
  Gain/1 -> Switch1/3  "OffSlewRate"
  En/1 -> Switch1/2, PumpOn/1
  Prevent div-by-zero/1 -> Math Function/1  "OnPeriod"
  Math Function/1 -> Switch1/1, Gain/1  "OnSlewRate"
  Constant1/1 -> Prevent div-by-zero/1

== system FuelSystemLibrary/Rem mass ==
  note: Rem Mass - calculation of remaining mass available in tank
      |
      | Revision History -
      | Issue 1.0 - ?? - SW - Initial Issue
      | Issue 1.1 - 28th October 2005 - DR - Added to FSP Generic Library
  Inst : Inport
  Demux4 : Demux  Outputs=20
  Gain : Gain  Gain=0.99  OutDataTypeStr=Inherit: Same as input  ParamDataTypeStr=Inherit: Same as input
  Product : Product  SaturateOnIntegerOverflow=on  OutDataTypeStr=Inherit: Same as first input
  Sum2 : Sum  Inputs=|+-  SaturateOnIntegerOverflow=on
  Temp2Density : FuelSystemLibrary/Temp2Density
  Terminator{1..15} (15 alike) : Terminator
  Mass : Outport
  wires:
  Demux4/12 -> Terminator3/1
  Gain/1 -> Mass/1
  Product/1 -> Gain/1
  Temp2Density/1 -> Product/2
  Sum2/1 -> Product/1
  Demux4/11 -> Terminator9/1
  Demux4/10 -> Terminator8/1
  Demux4/9 -> Terminator7/1
  Demux4/8 -> Temp2Density/3  "BValue"
  Demux4/7 -> Temp2Density/2  "AValue"
  Demux4/6 -> Temp2Density/1  "Temp"
  Demux4/5 -> Terminator2/1
  Demux4/4 -> Terminator1/1
  Demux4/3 -> Sum2/2  "Volume"
  Demux4/2 -> Terminator4/1  "Mass"
  Demux4/1 -> Sum2/1  "MaxVolume"
  Inst/1 -> Demux4/1
  Demux4/15 -> Terminator5/1
  Demux4/14 -> Terminator10/1
  Demux4/13 -> Terminator6/1
  Demux4/20 -> Terminator13/1
  Demux4/19 -> Terminator11/1
  Demux4/18 -> Terminator14/1
  Demux4/17 -> Terminator12/1
  Demux4/16 -> Terminator15/1

== system FuelSystemLibrary/RemMassV3 ==
  note: Rem Mass - calculation of remaining mass available in tank
      |
      | Revision History -
      | Issue 1.0 - 11th October 2012 Initial release
  Inst : Inport
  Demux4 : Demux  Outputs=22
  Gain : Gain  Gain=0.99  OutDataTypeStr=Inherit: Same as input  ParamDataTypeStr=Inherit: Same as input
  Product : Product  SaturateOnIntegerOverflow=on  OutDataTypeStr=Inherit: Same as first input
  Sum2 : Sum  Inputs=|+-  SaturateOnIntegerOverflow=on
  Temp2Density : FuelSystemLibrary/Temp2Density
  Terminator{1..17} (17 alike) : Terminator
  Mass : Outport
  wires:
  Demux4/16 -> Terminator15/1
  Demux4/17 -> Terminator12/1
  Demux4/18 -> Terminator14/1
  Demux4/19 -> Terminator11/1
  Demux4/20 -> Terminator13/1
  Demux4/13 -> Terminator6/1
  Demux4/14 -> Terminator10/1
  Demux4/15 -> Terminator5/1
  Inst/1 -> Demux4/1
  Demux4/1 -> Sum2/1  "MaxVolume"
  Demux4/2 -> Terminator4/1  "Mass"
  Demux4/3 -> Sum2/2  "Volume"
  Demux4/4 -> Terminator1/1
  Demux4/5 -> Terminator2/1
  Demux4/6 -> Temp2Density/1  "Temp"
  Demux4/7 -> Temp2Density/2  "AValue"
  Demux4/8 -> Temp2Density/3  "BValue"
  Demux4/9 -> Terminator7/1
  Demux4/10 -> Terminator8/1
  Demux4/11 -> Terminator9/1
  Sum2/1 -> Product/1
  Temp2Density/1 -> Product/2
  Product/1 -> Gain/1
  Gain/1 -> Mass/1
  Demux4/12 -> Terminator3/1
  Demux4/21 -> Terminator16/1
  Demux4/22 -> Terminator17/1

== system FuelSystemLibrary/Res ==
  note: Res - Resistor block
      |
      | Revision History -
      | Issue 1.0 - ?? - SW - Initial Issue
      | Issue 1.1 - 28th October 2005 - DR - Added to FSP Generic Library
  Constant2 : Constant  Value=PipeResistance
  Res : WrightSolverLib/Res
  Terminator3 : Terminator
  < : PMIOPort  Tag=PMCPort  Port=1  Side=Left
  > : PMIOPort  Tag=PMCPort  Port=2  Side=Right
  wires:
  Constant2/1 -> Res/1
  Res/1 -> Terminator3/1
  connections:
  Res/RConn1 -- >/RConn1
  </RConn1 -- Res/LConn1

== system FuelSystemLibrary/ResetNull ==
  note: Mass
  note: Temp
  note: ResetNull
      |
      | Revision History -
      | Issue 1.0 - ?? - SW - Initial Issue
      | Issue 1.1 - 28th October 2005 - DR - Added to FSP Generic Library
  Constant : Constant  Value=NoReset
  Constant1 : Constant  Value=NoReset
  Mux : Mux  Inputs=2
  Nul : Outport
  wires:
  Mux/1 -> Nul/1
  Constant/1 -> Mux/1
  Constant1/1 -> Mux/2

== system FuelSystemLibrary/RestrictorValve ==
  note: RestrictorValve - Used to for valves that need defined limits
      |
      | Revision History -
      | Issue 1.0 - ?? - SW - Initial Issue
      | Issue 1.1 - 28th October 2005 - DR - Added to FSP Generic Library
      | Issue 2.0 - 4th June 2010 - SW - WrightSolver version
  note: Orifice goes low-resistance
      | when valve open
  En : Inport
  C : Inport  Port=2
  Constant8 : Constant
  I Tap : WrightSolverLib/I Tap
  Oriface : FuelSystemLibrary/Oriface
  Switch4 : Switch  Threshold=DiscreteSwitchThreshold  SaturateOnIntegerOverflow=on  InputSameDT=on
  ValveHead : FuelSystemLibrary/ValveHead
  1P : PMIOPort  Tag=PMCPort  Port=1  Side=Left
  2P : PMIOPort  Tag=PMCPort  Port=2  Side=Right
  1BB : PMIOPort  Tag=PMCPort  Port=3  Side=Left
  2BB : PMIOPort  Tag=PMCPort  Port=4  Side=Right
  Stat : Outport
  wires:
  En/1 -> ValveHead/1
  I Tap/1 -> ValveHead/2  "Flow"
  ValveHead/2 -> [ValveConducting]
  ValveHead/1 -> Stat/1
  C/1 -> Switch4/3
  Constant8/1 -> Switch4/1
  [ValveConducting] -> Switch4/2
  Switch4/1 -> Oriface/1
  connections:
  1BB/RConn1 -- Oriface/LConn2
  Oriface/RConn2 -- 2BB/RConn1
  I Tap/RConn1 -- 2P/RConn1
  1P/RConn1 -- Oriface/LConn1
  Oriface/RConn1 -- I Tap/LConn1

== system FuelSystemLibrary/SinkAvail ==
  BBI1 : FuelSystemLibrary/BBI1
  BBSinkAvailOut : FuelSystemLibrary/BBSinkAvailOut
  In : PMIOPort  Tag=PMCPort  Port=1  Side=Left
  Out : PMIOPort  Tag=PMCPort  Port=2  Side=Right
  SinkA : Outport
  wires:
  BBI1/1 -> BBSinkAvailOut/1
  BBSinkAvailOut/1 -> SinkA/1
  connections:
  BBI1/RConn1 -- Out/RConn1
  In/RConn1 -- BBI1/LConn1

== system FuelSystemLibrary/SrcAvail ==
  BBI1 : FuelSystemLibrary/BBI1
  BBSrcAvailOut : FuelSystemLibrary/BBSrcAvailOut
  In : PMIOPort  Tag=PMCPort  Port=1  Side=Left
  Out : PMIOPort  Tag=PMCPort  Port=2  Side=Right
  SrcA : Outport
  wires:
  BBSrcAvailOut/1 -> SrcA/1
  BBI1/1 -> BBSrcAvailOut/1
  connections:
  In/RConn1 -- BBI1/LConn1
  BBI1/RConn1 -- Out/RConn1

== system FuelSystemLibrary/Supply ==
  note: NumInPlug - Plug for numerical interface to tank
      |
      | Revision History -
      | Issue 1.0 - ?? - SW - Initial Issue
      | Issue 1.1 - 28th October 2005 - DR - Added to FSP Generic Library
  BBTerm : FuelSystemLibrary/BBTerm
  Term : WrightSolverLib/Term
  1P : PMIOPort  Tag=PMCPort  Port=1  Side=Right
  1BB : PMIOPort  Tag=PMCPort  Port=2  Side=Right
  connections:
  BBTerm/LConn1 -- 1BB/RConn1
  Term/RConn1 -- 1P/RConn1

== system FuelSystemLibrary/Supply1 ==
  note: NumInPlug - Plug for numerical interface to tank
      |
      | Revision History -
      | Issue 1.0 - ?? - SW - Initial Issue
      | Issue 1.1 - 28th October 2005 - DR - Added to FSP Generic Library
  BBTerm : FuelSystemLibrary/BBTerm
  Term : WrightSolverLib/Term
  1P : PMIOPort  Tag=PMCPort  Port=1  Side=Right
  1BB : PMIOPort  Tag=PMCPort  Port=2  Side=Right
  connections:
  BBTerm/LConn1 -- 1BB/RConn1
  Term/RConn1 -- 1P/RConn1

== system FuelSystemLibrary/TJ1I2O ==
  BBBrk : FuelSystemLibrary/BBBrk
  BBBrk1 : FuelSystemLibrary/BBBrk1
  BBBrk2 : FuelSystemLibrary/BBBrk1
  I Tap : WrightSolverLib/I Tap
  I Tap1 : WrightSolverLib/I Tap
  I Tap2 : WrightSolverLib/I Tap
  PressTap1 : FuelSystemLibrary/PressTap
  TJIntersect : FuelSystemLibrary/TJIntersect
  TJLogic : FuelSystemLibrary/TJLogic
  1P : PMIOPort  Tag=PMCPort  Port=1  Side=Left
  1BB : PMIOPort  Tag=PMCPort  Port=2  Side=Left
  2P : PMIOPort  Tag=PMCPort  Port=3  Side=Right
  2BB : PMIOPort  Tag=PMCPort  Port=4  Side=Right
  3P : PMIOPort  Tag=PMCPort  Port=5  Side=Right
  3BB : PMIOPort  Tag=PMCPort  Port=6  Side=Right
  Inst : Outport
  wires:
  BBBrk/1 -> [BBIn3]
  [BBOut3] -> BBBrk/1
  [BBOut2] -> BBBrk2/1
  BBBrk2/1 -> [BBIn2]
  TJLogic/4 -> [BBOut3]
  TJLogic/3 -> [BBOut2]
  TJLogic/2 -> [BBOut1]
  [Flow3] -> TJLogic/7
  [Flow2] -> TJLogic/5
  [Flow1] -> TJLogic/3
  [BBOut1] -> BBBrk1/1
  BBBrk1/1 -> [BBIn1]
  I Tap/1 -> [Flow1]
  I Tap1/1 -> [Flow2]
  [BBIn1] -> TJLogic/2
  [BBIn2] -> TJLogic/4
  [BBIn3] -> TJLogic/6
  TJLogic/1 -> Inst/1
  PressTap1/1 -> TJLogic/1
  I Tap2/1 -> [Flow3]
  connections:
  1BB/RConn1 -- BBBrk1/RConn1
  2P/RConn1 -- I Tap1/LConn1
  2BB/RConn1 -- BBBrk2/RConn1
  I Tap1/RConn1 -- TJIntersect/LConn2
  1P/RConn1 -- I Tap/LConn1
  BBBrk/LConn1 -- 3BB/RConn1
  TJIntersect/RConn1 -- I Tap2/RConn1
  I Tap2/LConn1 -- 3P/RConn1
  PressTap1/RConn1 -- TJIntersect/LConn1
  I Tap/RConn1 -- PressTap1/LConn1

== system FuelSystemLibrary/TJ2I1O ==
  note: TJ2I10
      |
      | Revision History -
      | Issue 1.0 - ?? - SW - Initial Issue
      | Issue 1.1 - 28th October 2005 - DR - Added to FSP Generic Library
  BBBrk : FuelSystemLibrary/BBBrk
  BBBrk1 : FuelSystemLibrary/BBBrk1
  BBBrk2 : FuelSystemLibrary/BBBrk1
  I Tap : WrightSolverLib/I Tap
  I Tap1 : WrightSolverLib/I Tap
  I Tap2 : WrightSolverLib/I Tap
  PressTap : FuelSystemLibrary/PressTap
  TJIntersect : FuelSystemLibrary/TJIntersect
  TJLogic : FuelSystemLibrary/TJLogic
  1P : PMIOPort  Tag=PMCPort  Port=1  Side=Left
  1BB : PMIOPort  Tag=PMCPort  Port=2  Side=Left
  2P : PMIOPort  Tag=PMCPort  Port=3  Side=Left
  2BB : PMIOPort  Tag=PMCPort  Port=4  Side=Left
  3P : PMIOPort  Tag=PMCPort  Port=5  Side=Right
  3BB : PMIOPort  Tag=PMCPort  Port=6  Side=Right
  Inst : Outport
  wires:
  BBBrk/1 -> [BBIn3]
  [BBOut3] -> BBBrk/1
  [BBOut2] -> BBBrk2/1
  BBBrk2/1 -> [BBIn2]
  TJLogic/4 -> [BBOut3]
  TJLogic/3 -> [BBOut2]
  TJLogic/2 -> [BBOut1]
  [Flow3] -> TJLogic/7
  [Flow2] -> TJLogic/5
  [Flow1] -> TJLogic/3
  [BBOut1] -> BBBrk1/1
  BBBrk1/1 -> [BBIn1]
  I Tap/1 -> [Flow1]
  I Tap1/1 -> [Flow2]
  [BBIn1] -> TJLogic/2
  [BBIn2] -> TJLogic/4
  [BBIn3] -> TJLogic/6
  TJLogic/1 -> Inst/1
  PressTap/1 -> TJLogic/1
  I Tap2/1 -> [Flow3]
  connections:
  BBBrk/LConn1 -- 3BB/RConn1
  2BB/RConn1 -- BBBrk2/RConn1
  1BB/RConn1 -- BBBrk1/RConn1
  I Tap1/RConn1 -- TJIntersect/LConn2
  I Tap/RConn1 -- TJIntersect/LConn1
  2P/RConn1 -- I Tap1/LConn1
  1P/RConn1 -- I Tap/LConn1
  TJIntersect/RConn1 -- PressTap/LConn1
  I Tap2/LConn1 -- 3P/RConn1
  PressTap/RConn1 -- I Tap2/RConn1

== system FuelSystemLibrary/TJFan ==
  note: Special TJ, breaking
      | cross dependancy
      | between Ports 1/2
  BBBrk : FuelSystemLibrary/BBBrk
  BBBrk1 : FuelSystemLibrary/BBBrk1
  BBBrk2 : FuelSystemLibrary/BBBrk1
  Fan : WrightSolverLib/Fan
  I Tap : WrightSolverLib/I Tap
  I Tap1 : WrightSolverLib/I Tap
  I Tap2 : WrightSolverLib/I Tap
  PressTap : FuelSystemLibrary/PressTap
  TJFanLogic : FuelSystemLibrary/TJFanLogic
  1P : PMIOPort  Tag=PMCPort  Port=1  Side=Left
  1BB : PMIOPort  Tag=PMCPort  Port=2  Side=Left
  2P : PMIOPort  Tag=PMCPort  Port=3  Side=Left
  2BB : PMIOPort  Tag=PMCPort  Port=4  Side=Left
  3P : PMIOPort  Tag=PMCPort  Port=5  Side=Right
  3BB : PMIOPort  Tag=PMCPort  Port=6  Side=Right
  Inst : Outport
  wires:
  BBBrk/1 -> [BBIn3]
  [BBOut3] -> BBBrk/1
  [BBOut2] -> BBBrk2/1
  BBBrk2/1 -> [BBIn2]
  TJFanLogic/4 -> [BBOut3]
  TJFanLogic/3 -> [BBOut2]
  TJFanLogic/2 -> [BBOut1]
  [Flow3] -> TJFanLogic/7
  [Flow2] -> TJFanLogic/5
  [Flow1] -> TJFanLogic/3
  [BBOut1] -> BBBrk1/1
  BBBrk1/1 -> [BBIn1]
  I Tap/1 -> [Flow1]
  I Tap1/1 -> [Flow2]
  [BBIn1] -> TJFanLogic/2
  [BBIn2] -> TJFanLogic/4
  [BBIn3] -> TJFanLogic/6
  TJFanLogic/1 -> Inst/1
  [Press] -> TJFanLogic/1
  PressTap/1 -> [Press]
  I Tap2/1 -> [Flow3]
  connections:
  BBBrk/LConn1 -- 3BB/RConn1
  2BB/RConn1 -- BBBrk2/RConn1
  1BB/RConn1 -- BBBrk1/RConn1
  I Tap1/RConn1 -- Fan/LConn2
  I Tap/RConn1 -- Fan/LConn1
  2P/RConn1 -- I Tap1/LConn1
  1P/RConn1 -- I Tap/LConn1
  Fan/RConn1 -- PressTap/LConn1
  I Tap2/LConn1 -- 3P/RConn1
  PressTap/RConn1 -- I Tap2/RConn1
